simulink model "lab6_uncontrolled3phasefullwave"  (R2021b)
settings: Solver=VariableStepAuto  StartTime=0.0  StopTime=0.1  RelTol=1e-3
libraries: spsDiodeLib x6, spsACVoltageSourceLib x3, spsCurrentMeasurementLib x1, spsGroundLib x1, spsRMSLib x1, spsSeriesRLCBranchLib x1, spsThreePhaseVIMeasurementLib x1, spsVoltageMeasurementLib x1, spspowerguiLib x1
settings Model: Creator=Petulla  LastModifiedBy=Asus
settings SolverCC: AlgebraicLoopSolver=TrustRegion

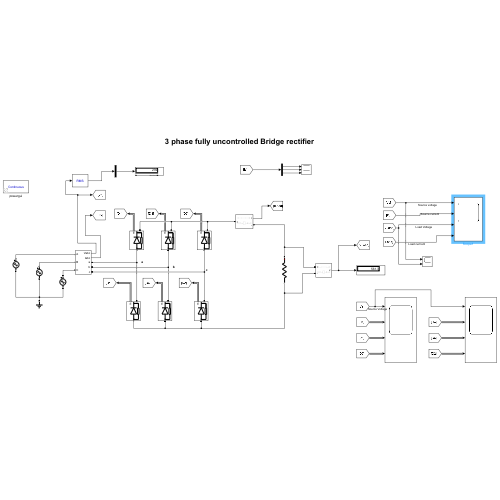
[thumbnail: Simulink's stored preview of the top-level diagram]
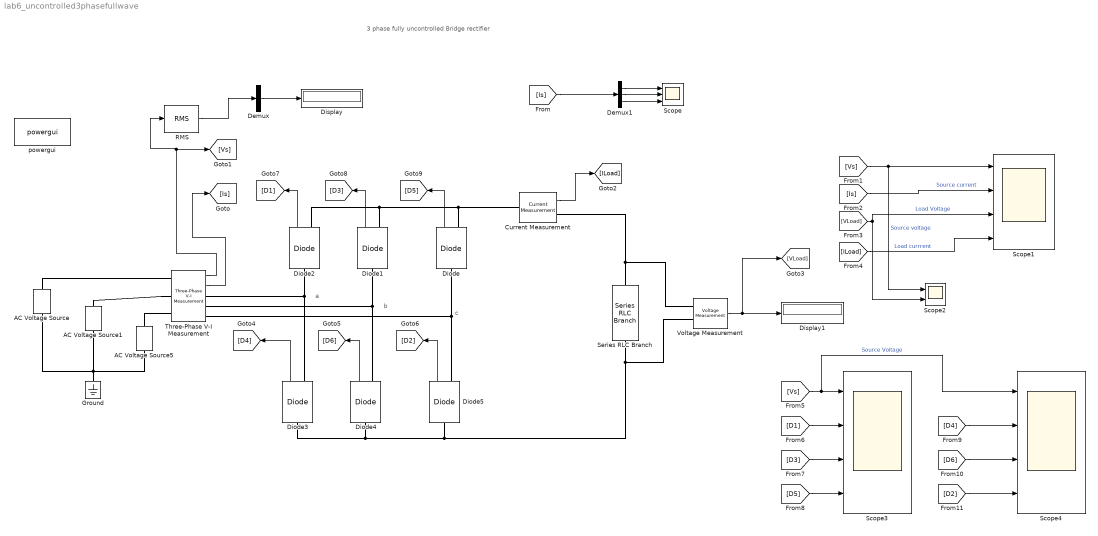
== system lab6_uncontrolled3phasefullwave ==
  note: a
  note: 3 phase fully uncontrolled Bridge rectifier
  note: b
  note: c
  AC Voltage Source : spsACVoltageSourceLib/AC Voltage Source  Amplitude=230*sqrt(2)  Phase=0  Frequency=50  SampleTime=0  Measurements=None  BusType=swing  Pref=10e3  Qref=0  Qmin=-inf  Qmax=+inf
  AC Voltage Source1 : spsACVoltageSourceLib/AC Voltage Source  Amplitude=230*sqrt(2)  Phase=-120  Frequency=50  SampleTime=0  Measurements=None  BusType=swing  Pref=10e3  Qref=0  Qmin=-inf  Qmax=+inf
  AC Voltage Source5 : spsACVoltageSourceLib/AC Voltage Source  Amplitude=230*sqrt(2)  Phase=120  Frequency=50  SampleTime=0  Measurements=None  BusType=swing  Pref=10e3  Qref=0  Qmin=-inf  Qmax=+inf
  Current Measurement : spsCurrentMeasurementLib/Current Measurement  PhasorSimulation=off  OutputType=Complex  PSBequivalent=0
  Demux : Demux  Outputs=1
  Demux1 : Demux  Outputs=3
  Diode{,1..5} (6 alike) : spsDiodeLib/Diode  Ron=0.001  Lon=0  Vf=0.8  IC=0  UseSnubber=0  Rs=500  Cs=250e-9  Measurements=on
  Display : Display
  Display1 : Display
  Ground : spsGroundLib/Ground  LConnTagsString=a
  RMS : spsRMSLib/RMS  TrueRMS=on  Freq=60  RMSInit=230  Ts=0
  Scope : Scope  NumInputPorts=3
  Scope1 : Scope  NumInputPorts=4
  Scope2 : Scope  NumInputPorts=2
  Scope3 : Scope  NumInputPorts=4
  Scope4 : Scope  NumInputPorts=4
  Series RLC Branch : spsSeriesRLCBranchLib/Series RLC Branch  LConnTagsString=__new0  RConnTagsString=__new0  BranchType=R  Resistance=2.5  Inductance=4.5e-3  SetiL0=off  InitialCurrent=0  Capacitance=1e-6  Setx0=off  InitialVoltage=0  Measurements=Branch current
  Three-Phase V-I Measurement : spsThreePhaseVIMeasurementLib/Three-Phase V-I Measurement  VoltageMeasurement=phase-to-ground  SetLabelV=off  LabelV=Vabc  Vpu=off  VpuLL=off  CurrentMeasurement=yes  SetLabelI=off  LabelI=Iabc  Ipu=off  Pbase=100e6  Vbase=500e3  OutputType=Complex  PhasorSimulation=off  PSBequivalent=0
  Voltage Measurement : spsVoltageMeasurementLib/Voltage Measurement  PhasorSimulation=off  OutputType=Complex  PSBequivalent=0
  powergui : spspowerguiLib/powergui  Priority=1  SimulationMode=Continuous  SampleTime=50e-6  frequency=60  Iterations=50  frequencyindice=50  Pbase=100e6  ErrMax=1e-4  UnitsV=kV  UnitsW=MW  buscounter=0  FunctionMessages=off  echomessages=off  EnableUseOfTLC=off  CurrentSourceSwitches=off  DisableSnubberDevices=off  DisableRonSwitches=off  DisableVfSwitches=off  DisplayEquations=off  AutomaticDiscreteSolvers=off  SolverType=Tustin/Backward Euler (TBE)  Interpol=off  ExternalGateDelay=off  methode=off  Ts=100  x0status=blocks  SPID=on  SwTol=0  HookPort=off  NonlinearTolerance=1e-4  nMaxIteration=100  ContinueOnMaxIteration=off  RestoreLinks=warning  ResistiveCurrentMeasurement=off  Frange=[0:2:500]  Ylog=off  Xlog=on  ShowGrid=off  save=off  variable=ZData  structure=0  ZoomFFT=off  StartTime=0.0  cycles=1  DisplayStyle=1  fundamental=60  FreqAxis=off  MaxFrequency=1000  frequencyindicesteady=1  RmsSteady=1  display=off
  wires:
  Three-Phase V-I Measurement/2 -> [Is]
  Three-Phase V-I Measurement/1 -> RMS/1, [Vs]
  Current Measurement/1 -> [ILoad]
  Voltage Measurement/1 -> [VLoad], Display1/1
  [Is] -> Demux1/1
  Demux1/1 -> Scope/1
  Demux1/2 -> Scope/2
  Demux1/3 -> Scope/3
  [Vs] -> Scope2/1, Scope1/1  "Source voltage"
  [Is] -> Scope1/2  "Source current"
  [VLoad] -> Scope2/2, Scope1/3  "Load Voltage"
  [ILoad] -> Scope1/4  "Load currrent"
  Demux/1 -> Display/1
  RMS/1 -> Demux/1
  Diode3/1 -> [D4]
  Diode4/1 -> [D6]
  Diode5/1 -> [D2]
  Diode2/1 -> [D1]
  Diode1/1 -> [D3]
  Diode/1 -> [D5]
  [Vs] -> Scope4/1, Scope3/1  "Source Voltage"
  [D1] -> Scope3/2
  [D3] -> Scope3/3
  [D5] -> Scope3/4
  [D2] -> Scope4/4
  [D6] -> Scope4/3
  [D4] -> Scope4/2
  connections:
  Current Measurement/LConn1 -- Diode2/RConn1 -- Diode1/RConn1 -- Diode/RConn1
  Current Measurement/RConn1 -- Voltage Measurement/LConn1 -- Series RLC Branch/LConn1
  Series RLC Branch/RConn1 -- Diode4/LConn1 -- Diode3/LConn1 -- Diode5/LConn1 -- Voltage Measurement/LConn2
  Diode3/RConn1 -- Three-Phase V-I Measurement/RConn1 -- Diode2/LConn1
  Diode4/RConn1 -- Three-Phase V-I Measurement/RConn2 -- Diode1/LConn1
  Diode5/RConn1 -- Three-Phase V-I Measurement/RConn3 -- Diode/LConn1
  Three-Phase V-I Measurement/LConn2 -- AC Voltage Source1/RConn1
  AC Voltage Source5/RConn1 -- Three-Phase V-I Measurement/LConn3
  AC Voltage Source/RConn1 -- Three-Phase V-I Measurement/LConn1
  AC Voltage Source5/LConn1 -- AC Voltage Source/LConn1 -- AC Voltage Source1/LConn1 -- Ground/LConn1
